simulink model "MicrogridControl"  (R2025b)
settings: Solver=VariableStepAuto  StartTime=0.0  StopTime=8  FixedStep=Ts  RelTol=1e-3
PreLoadFcn:
  | NormalOperation;
  | MicrogridControlParam;
undefined symbols (not defined in the file): base, bessModeInitial, bessSystem, bessVoltage, breakerStatus, DiscIntNeverNeededParam, ee_sli_rtmsupport, event, gcbh, generator, gflInverter, gfmInverter, Inertia, lineInductance, lineResistance, machine, plannedIsland, pmsm, powerLimit, powerQuality, PV, PVInverter, ref, resync, solar, solarInsolationChange, systemFrequency, Ts, windController, windSystem, windTurbine
libraries: nesl_utility x234, ee_lib x174, fl_lib x143, eeGeneralControl x137, simulink x78, eeTransforms x47, slpidlib x23, nesl_utility_internal x12, eePwmGenerator x9, eeSinusoidalMeasurementV2 x9, custom_lib x7, batteryecm_lib x6
(part 3 of 25)

== system MicrogridControl/Solar ==
  Constant1 : Constant  Value=298
  Constant2 : Constant  Value=0
  Constant3 : Constant  Value=0
  Constant4 : Constant
  Solar Plant Integrated : Subsystem  Variant=on  VariantControlMode=label  LabelModeActiveChoice=Detailed  mask(Solar){fidelity=Detailed, plantRating=PV.plantRating, Vac=PV.Vac, frequency=PV.frequency, iMaxPU=PVInverter.iMaxPU, efficiency=PV.converterEfficiency, baseVoltageDC=PV.baseVoltageDC, nParallel=112, nSeries=30, capacitance=PVInverter.capacitance, filterInductance=PVInverter.filterInductance, filterResistance=PVInverter.filterResistance, panelType=Poly-crystalline, panelRating=PV.panelRating, Isc=PV.Isc, Voc=PV.Voc, irradianceSTC=PV.irradianceSTC, temperatureSTC=PV.temperatureSTC, alpha=PV.alpha, beta=PV.beta, mode=Maximum power point tracking, converterFidelity=Average, fSw=PV.switchingFrequency}
      mask prompts: fidelity "Modeling Option"; plantRating "Solar Plant Rating (kW)"; Vac "Rated AC side voltage (phase-phase RMS) (V)"; frequency "Rated electrical frequency at AC side (Hz)"; iMaxPU "Maximum converter current (pu)"; efficiency "Converter Efficiency (%)"; baseVoltageDC "Voltage on DC side (V)"; nParallel "Number of panels in parallel"; nSeries "Number of panels in series"; capacitance "DC bus capacitance (F)"; filterInductance "Filter inductance (H)"; filterResistance "Filter series resistance (Ohm)"; panelType "Panel Type"; panelRating "Panel Rating (W)"; Isc "Short-circuit current (A)"; Voc "Open-circuit voltage (V)"; irradianceSTC "Irradiance at STC (W/m² )"; temperatureSTC "Temperature at STC (°K)"; alpha "Temperature co-efficient for current (A/°K)"; beta "Temperature co-efficient for voltage (V/°K)"; mode "Operating Mode"; converterFidelity "Converter Fidelity"; fSw "Switching Frequency (kHz)"
      mask help: This block models a Solar PV plant. The detailed variant models MPPT, voltage and current controllers. The simplified variant is based on Anderson's translational equations. Select simplified mode for faster simulation using fixed efficiency and rated power.
      settings: CopyFcn=set_param(gcbh,'LinkStatus','none');
      mask Help: web('SolarPlant.html')
      mask TypeOptions fidelity: Detailed | Simplified
      mask Callback fidelity: component.mask.fidelitySelection;
      mask TypeOptions nParallel: Detailed/PV Plant & Controller/PV Plant/nParallel
      mask TypeOptions nSeries: Detailed/PV Plant & Controller/PV Plant/nSeries
      mask TypeOptions panelType: Poly-crystalline | Mono-crystalline | Cadmium-Telluride | Others
      mask Callback panelType: component.mask.selectSolarPanelType;
      mask TypeOptions mode: Maximum power point tracking | Power reference
      mask Callback mode:
      | % choice = get_param(gcb,'mode');
      | % blockPath = [gcb,'/','Solar','/','Simplified','/','Solar_Plant'];
      | % blockHandle = get_param(blockPath, 'Handle');
      | % if strcmp(choice,'Maximum power point tracking')
      | %     set_param(blockPath,'modelling_option','ModellingOption.maximumPower');
      | % else
      | %     set_param(blockPath,'modelling_option','ModellingOption.powerReference');
      | % end
      mask TypeOptions converterFidelity: Detailed/PV Plant & Controller/PV Plant/converterFidelity
      mask Callback converterFidelity: component.mask.setSwitchingFrequency;
      mask TypeOptions fSw: Detailed/PV Plant & Controller/PV Plant/fSw
      mask DialogControl generalDetailed Prompt: General
      mask DialogControl cellDetailed Prompt: Solar Cell
      mask DialogControl partsCatalog Prompt: Click to choose from parts catalog
      mask DialogControl partsCatalog Callback: component.mask.openParamManager;
      mask DialogControl panelCalculation Prompt: Calculate number of panels
      mask DialogControl panelCalculation Callback: component.mask.setPanelNumber;
      mask DialogControl configureSolarCell Prompt: Edit Solar Cell Parameters
      mask DialogControl configureSolarCell Callback:
      | blockPath = [gcb,'/','Detailed','/','PV Plant & Controller','/','PV Plant','/','PV Array'];
      |     component.mask.openBlock(blockPath);
      mask DialogControl controllerDetailed Prompt: Solar PV Controller
      mask DialogControl configurePVController Prompt: Edit MPPT Controller
      mask DialogControl configurePVController Callback:
      | blockPath = [gcb,'/','Detailed','/','PV Plant & Controller','/','Controller','/','MPPT','/','Solar PV Controller'];
      |     component.mask.openBlock(blockPath);
      mask DialogControl configurePRefControl Prompt: Edit Power Reference Controller
      mask DialogControl configurePRefControl Callback:
      | blockPath = [gcb,'/','Detailed','/','PV Plant & Controller','/','Controller','/','Power Reference','/','Power Reference Controller'];
      |     component.mask.openBlock(blockPath);
      mask DialogControl cellSimplified Prompt: Solar Cell
      mask DialogControl converter Prompt: Converter
      mask DialogControl editConverter Prompt: Edit converter parameters
      mask DialogControl editConverter Callback:
      | converterFidelity = get_param(gcb,'converterFidelity');
      | blockPath = [gcb,'/','Detailed','/','PV Plant & Controller','/','PV Plant','/','Converter','/',converterFidelity,'/','Converter'];
      | component.mask.openBlock(blockPath);
      mask Display: image('solarPlant.png');
  Solar Plant Integrated1 : Subsystem  Variant=on  VariantControlMode=label  LabelModeActiveChoice=Detailed  mask(Solar){fidelity=Detailed, plantRating=PV.plantRating, Vac=PV.Vac, frequency=PV.frequency, iMaxPU=PVInverter.iMaxPU, efficiency=PV.converterEfficiency, baseVoltageDC=PV.baseVoltageDC, nParallel=112, nSeries=30, capacitance=PVInverter.capacitance, filterInductance=PVInverter.filterInductance, filterResistance=PVInverter.filterResistance, panelType=Poly-crystalline, panelRating=PV.panelRating, Isc=PV.Isc, Voc=PV.Voc, irradianceSTC=PV.irradianceSTC, temperatureSTC=PV.temperatureSTC, alpha=PV.alpha, beta=PV.beta, mode=Maximum power point tracking, converterFidelity=Average, fSw=PV.switchingFrequency}
      mask prompts: fidelity "Modeling Option"; plantRating "Solar Plant Rating (kW)"; Vac "Rated AC side voltage (phase-phase RMS) (V)"; frequency "Rated electrical frequency at AC side (Hz)"; iMaxPU "Maximum converter current (pu)"; efficiency "Converter Efficiency (%)"; baseVoltageDC "Voltage on DC side (V)"; nParallel "Number of panels in parallel"; nSeries "Number of panels in series"; capacitance "DC bus capacitance (F)"; filterInductance "Filter inductance (H)"; filterResistance "Filter series resistance (Ohm)"; panelType "Panel Type"; panelRating "Panel Rating (W)"; Isc "Short-circuit current (A)"; Voc "Open-circuit voltage (V)"; irradianceSTC "Irradiance at STC (W/m² )"; temperatureSTC "Temperature at STC (°K)"; alpha "Temperature co-efficient for current (A/°K)"; beta "Temperature co-efficient for voltage (V/°K)"; mode "Operating Mode"; converterFidelity "Converter Fidelity"; fSw "Switching Frequency (kHz)"
      mask help: This block models a Solar PV plant. The detailed variant models MPPT, voltage and current controllers. The simplified variant is based on Anderson's translational equations. Select simplified mode for faster simulation using fixed efficiency and rated power.
      settings: CopyFcn=set_param(gcbh,'LinkStatus','none');
      mask Help: web('SolarPlant.html')
      mask TypeOptions fidelity: Detailed | Simplified
      mask Callback fidelity: component.mask.fidelitySelection;
      mask TypeOptions nParallel: Detailed/PV Plant & Controller/PV Plant/nParallel
      mask TypeOptions nSeries: Detailed/PV Plant & Controller/PV Plant/nSeries
      mask TypeOptions panelType: Poly-crystalline | Mono-crystalline | Cadmium-Telluride | Others
      mask Callback panelType: component.mask.selectSolarPanelType;
      mask TypeOptions mode: Maximum power point tracking | Power reference
      mask Callback mode:
      | % choice = get_param(gcb,'mode');
      | % blockPath = [gcb,'/','Solar','/','Simplified','/','Solar_Plant'];
      | % blockHandle = get_param(blockPath, 'Handle');
      | % if strcmp(choice,'Maximum power point tracking')
      | %     set_param(blockPath,'modelling_option','ModellingOption.maximumPower');
      | % else
      | %     set_param(blockPath,'modelling_option','ModellingOption.powerReference');
      | % end
      mask TypeOptions converterFidelity: Detailed/PV Plant & Controller/PV Plant/converterFidelity
      mask Callback converterFidelity: component.mask.setSwitchingFrequency;
      mask TypeOptions fSw: Detailed/PV Plant & Controller/PV Plant/fSw
      mask DialogControl generalDetailed Prompt: General
      mask DialogControl cellDetailed Prompt: Solar Cell
      mask DialogControl partsCatalog Prompt: Click to choose from parts catalog
      mask DialogControl partsCatalog Callback: component.mask.openParamManager;
      mask DialogControl panelCalculation Prompt: Calculate number of panels
      mask DialogControl panelCalculation Callback: component.mask.setPanelNumber;
      mask DialogControl configureSolarCell Prompt: Edit Solar Cell Parameters
      mask DialogControl configureSolarCell Callback:
      | blockPath = [gcb,'/','Detailed','/','PV Plant & Controller','/','PV Plant','/','PV Array'];
      |     component.mask.openBlock(blockPath);
      mask DialogControl controllerDetailed Prompt: Solar PV Controller
      mask DialogControl configurePVController Prompt: Edit MPPT Controller
      mask DialogControl configurePVController Callback:
      | blockPath = [gcb,'/','Detailed','/','PV Plant & Controller','/','Controller','/','MPPT','/','Solar PV Controller'];
      |     component.mask.openBlock(blockPath);
      mask DialogControl configurePRefControl Prompt: Edit Power Reference Controller
      mask DialogControl configurePRefControl Callback:
      | blockPath = [gcb,'/','Detailed','/','PV Plant & Controller','/','Controller','/','Power Reference','/','Power Reference Controller'];
      |     component.mask.openBlock(blockPath);
      mask DialogControl cellSimplified Prompt: Solar Cell
      mask DialogControl converter Prompt: Converter
      mask DialogControl editConverter Prompt: Edit converter parameters
      mask DialogControl editConverter Callback:
      | converterFidelity = get_param(gcb,'converterFidelity');
      | blockPath = [gcb,'/','Detailed','/','PV Plant & Controller','/','PV Plant','/','Converter','/',converterFidelity,'/','Converter'];
      | component.mask.openBlock(blockPath);
      mask Display: image('solarPlant.png');
  Step1 : Step  Time=solarInsolationChange  Before=1000  After=800  SampleTime=0
  Transformer : Subsystem  Variant=on  VariantControlMode=label  LabelModeActiveChoice=Detailed  mask{fidelity=Detailed}
      mask prompts: fidelity "Modeling Option"
      mask TypeOptions fidelity: Detailed | Simplified
      mask Callback fidelity:
      | choice = get_param(gcb,'fidelity');
      | switch choice
      |     case 'Detailed'
      |         set_param(gcb, 'LabelModeActiveChoice', 'Detailed');
      |     case 'Simplified'
      |          set_param(gcb, 'LabelModeActiveChoice', 'Simplified');
      |     otherwise
      |         disp('Choose proper variant');
      | end
  Transformer1 : Subsystem  Variant=on  VariantControlMode=label  LabelModeActiveChoice=Detailed  mask{fidelity=Detailed}
      mask prompts: fidelity "Modeling Option"
      mask TypeOptions fidelity: Detailed | Simplified
      mask Callback fidelity:
      | choice = get_param(gcb,'fidelity');
      | switch choice
      |     case 'Detailed'
      |         set_param(gcb, 'LabelModeActiveChoice', 'Detailed');
      |     case 'Simplified'
      |          set_param(gcb, 'LabelModeActiveChoice', 'Simplified');
      |     otherwise
      |         disp('Choose proper variant');
      | end
  ~ : PMIOPort  Side=Left
  wires:
  Constant1/1 -> Solar Plant Integrated1/2(T), Solar Plant Integrated/2(T)
  Constant4/1 -> Solar Plant Integrated1/5(Mode), Solar Plant Integrated/5(Mode)
  Constant2/1 -> Solar Plant Integrated1/3(Pref), Solar Plant Integrated/3(Pref)
  Constant3/1 -> Solar Plant Integrated1/4(Qref), Solar Plant Integrated/4(Qref)
  Step1/1 -> Solar Plant Integrated1/1(Ir), Solar Plant Integrated/1(Ir)
  connections:
  Transformer/RConn1 -- Transformer1/RConn1 -- ~/RConn1
  Solar Plant Integrated/RConn1 -- Transformer/LConn1
  Solar Plant Integrated1/RConn1 -- Transformer1/LConn1

== system MicrogridControl/Subsystem ==
  Subsystem1 : Subsystem
      settings: PortSchema="{\"entries\":[{\"content\":{\"sides\":[{\"content\":{\"connectorIds\":[\"LConn1\"]},\"type\":\"ConnectorPlacement.EquallySpacedRectSide\",\"uuid\":\"0c8863a2-a78f-4a73-a820-c6aa5bdc2133\"},{\"content\":{\"connectorIds\":[\"RConn1\"],\"side\":\"RIGHT\"},\"type\":\"ConnectorPlacement.EquallySpacedRectSide\",\"uuid\":\"2028a368-e468-46fb-8c3f-9ce74e7f0a45\"},{\"content\":{\"side\":\"TOP\"},\"type\":\"ConnectorPlacement.EquallySpacedRectSide\",\"uuid\":\"1b144116-ac84-43c3-ac53-ab33c5b71658\"},{\"content\":{\"connectorIds\":[\"Out1\",\"Out2\"],\"side\":\"BOTTOM\"},\"type\":\"ConnectorPlacement.EquallySpacedRectSide\",\"uuid\":\"3e4d0e65-8f44-4e57-8d60-68941db834c2\"}]},\"type\":\"ConnectorPlacement.EquallySpacedConnector\",\"uuid\":\"a27c8f54-ed82-4619-aed8-d6cf5e2c28e1\"}],\"packageUris\":[\"http://schema.mathworks.com/mf0/Connector/R2020b\"],\"version\":\"1.0\"}"
      mask Display: image('measurements.png');
  Conn1 : PMIOPort  Side=Left
  Conn2 : PMIOPort  Port=2  Side=Right
  Bus Element Out : Outport  PortName=Solar  Element=P
  BusElementOut : Outport  PortName=Solar  Element=Q
  wires:
  Subsystem1/2(P) -> Bus Element Out/1  "Solar"
  Subsystem1/1(Q) -> BusElementOut/1  "Solar"
  connections:
  Conn1/RConn1 -- Subsystem1/RConn1
  Subsystem1/LConn1 -- Conn2/RConn1

== system MicrogridControl/Subsystem1 ==
  Circuit Breaker : Subsystem
  Constant : Constant  Value=breakerStatus.generator
  Subsystem9 : Subsystem
      settings: PortSchema="{\"entries\":[{\"content\":{\"sides\":[{\"content\":{\"connectorIds\":[\"LConn1\"]},\"type\":\"ConnectorPlacement.EquallySpacedRectSide\",\"uuid\":\"0c8863a2-a78f-4a73-a820-c6aa5bdc2133\"},{\"content\":{\"connectorIds\":[\"RConn1\"],\"side\":\"RIGHT\"},\"type\":\"ConnectorPlacement.EquallySpacedRectSide\",\"uuid\":\"2028a368-e468-46fb-8c3f-9ce74e7f0a45\"},{\"content\":{\"side\":\"TOP\"},\"type\":\"ConnectorPlacement.EquallySpacedRectSide\",\"uuid\":\"1b144116-ac84-43c3-ac53-ab33c5b71658\"},{\"content\":{\"connectorIds\":[\"Out1\",\"Out2\"],\"side\":\"BOTTOM\"},\"type\":\"ConnectorPlacement.EquallySpacedRectSide\",\"uuid\":\"3e4d0e65-8f44-4e57-8d60-68941db834c2\"}]},\"type\":\"ConnectorPlacement.EquallySpacedConnector\",\"uuid\":\"a27c8f54-ed82-4619-aed8-d6cf5e2c28e1\"}],\"packageUris\":[\"http://schema.mathworks.com/mf0/Connector/R2020b\"],\"version\":\"1.0\"}"
      mask Display: image('measurements.png');
  ~ : PMIOPort  Side=Left
  Conn2 : PMIOPort  Port=2  Side=Right
  Bus Element Out : Outport  PortName=Generator  Element=P
  BusElementOut : Outport  PortName=Generator  Element=Q
  wires:
  Subsystem9/2(P) -> Bus Element Out/1  "Diesel"
  Subsystem9/1(Q) -> BusElementOut/1  "Diesel"
  Constant/1 -> Circuit Breaker/1(BRK)
  connections:
  ~/RConn1 -- Circuit Breaker/LConn1
  Subsystem9/RConn1 -- Circuit Breaker/RConn1
  Conn2/RConn1 -- Subsystem9/LConn1

== system MicrogridControl/Subsystem10 ==
  In : PMIOPort  Side=Left
  Out : PMIOPort  Port=2  Side=Right
  connections:
  Out/RConn1 -- In/RConn1

== system MicrogridControl/Subsystem12 ==
  RLC (Three-Phase) : ee_lib/Passive/RLC Assemblies/RLC (Three-Phase)  port_option=ee.enum.threePhasePort.composite  component_structure=ee.enum.rlc.structure.SeriesRL  R=1e-2*10 Ohm  L=1e-6*10 H  C=1e-6 F  R_parasitic=0 Ohm  G_parasitic=0 1/Ohm  IL_specify=on  IL_priority=None  IL=[0, 0, 0] A  IL_nominal_specify=off  IL_nominal_value=1  IL_nominal_unit=A  VC_specify=off  VC_priority=High  VC=[0, 0, 0] V  VC_nominal_specify=off  VC_nominal_value=1  VC_nominal_unit=V
      settings: InternalSimscapePortConfiguration="{\"Bottom\":[],\"Left\":[{\"id\":\"N1\",\"label\":\"~1\",\"type\":\"foundation.electrical.three_phase\"}],\"Right\":[{\"id\":\"N2\",\"label\":\"~2\",\"type\":\"foundation.electrical.three_phase\"}],\"Top\":[]}"
  In : PMIOPort  Side=Left
  Out : PMIOPort  Port=2  Side=Right
  connections:
  RLC (Three-Phase)/LConn1 -- In/RConn1
  RLC (Three-Phase)/RConn1 -- Out/RConn1

== system MicrogridControl/Subsystem13 ==
  Electrical Reference : fl_lib/Electrical/Electrical Elements/Electrical Reference  Commented=on
  Subsystem : Subsystem
      settings: PortSchema="{\"entries\":[{\"content\":{\"sides\":[{\"content\":{\"connectorIds\":[\"LConn1\"]},\"type\":\"ConnectorPlacement.EquallySpacedRectSide\",\"uuid\":\"0c8863a2-a78f-4a73-a820-c6aa5bdc2133\"},{\"content\":{\"connectorIds\":[\"RConn1\"],\"side\":\"RIGHT\"},\"type\":\"ConnectorPlacement.EquallySpacedRectSide\",\"uuid\":\"2028a368-e468-46fb-8c3f-9ce74e7f0a45\"},{\"content\":{\"side\":\"TOP\"},\"type\":\"ConnectorPlacement.EquallySpacedRectSide\",\"uuid\":\"1b144116-ac84-43c3-ac53-ab33c5b71658\"},{\"content\":{\"connectorIds\":[\"Out1\",\"Out2\"],\"side\":\"BOTTOM\"},\"type\":\"ConnectorPlacement.EquallySpacedRectSide\",\"uuid\":\"3e4d0e65-8f44-4e57-8d60-68941db834c2\"}]},\"type\":\"ConnectorPlacement.EquallySpacedConnector\",\"uuid\":\"a27c8f54-ed82-4619-aed8-d6cf5e2c28e1\"}],\"packageUris\":[\"http://schema.mathworks.com/mf0/Connector/R2020b\"],\"version\":\"1.0\"}"
      mask Display: image('measurements.png');
  Two-Winding Transformer (Three-Phase)1 : ee_lib/Passive/Transformers/Two-Winding Transformer (Three-Phase)  Commented=on  SRated=5e6 A*V  FRated=60 Hz  Winding1Connection=ee.enum.windingconnection.Yg  VRated1=11000 V  Winding2Connection=ee.enum.windingconnection.Yg  VRated2=4160 V  CoreType=ee.enum.coretype.threelimb  pu_Rw1=0.01  pu_Rw2=0.01  leakage_reactance_option=ee.enum.transformer_leakage.include  pu_Xl1=0.05  pu_Xl2=0.05  magnetizing_resistance_option=ee.enum.transformer_magnetizingResistance.exclude  pu_Rm=500  magnetizing_reactance_option=ee.enum.transformer_magnetizingReactance.exclude  saturation_option=ee.enum.transformer_saturation.exclude  pu_Xm=500  current_data=[0, .002, 1, 2]  magnetic_flux_data=[0, 1.2, 1.5, 1.51]  pu_X0=0.5  i1_specify=off  i1_priority=None  i1=[0, 0, 0] A  i1_nominal_specify=off  i1_nominal_value=1  i1_nominal_unit=A  i2_specify=off  i2_priority=None  i2=[0, 0, 0] A  i2_nominal_specify=off  i2_nominal_value=1  i2_nominal_unit=A  phi_specify=off  phi_priority=None  phi=[0, 0, 0]  phi_nominal_specify=off  phi_nominal_value=1  phi_nominal_unit=1  power_dissipated_specify=off  power_dissipated_priority=None  power_dissipated=0 W  power_dissipated_nominal_specify=off  power_dissipated_nominal_value=1  power_dissipated_nominal_unit=W
      settings: InternalSimscapePortConfiguration="{\"Bottom\":[],\"Left\":[{\"id\":\"N1\",\"label\":\"~1\",\"type\":\"foundation.electrical.three_phase\"}],\"Right\":[{\"id\":\"N2\",\"label\":\"~2\",\"type\":\"foundation.electrical.three_phase\"}],\"Top\":[]}"
  Wye-Connected Load : ee_lib/Passive/RLC Assemblies/Wye-Connected Load  Commented=on  port_option=ee.enum.threePhasePort.composite  parameterization=ee.enum.rlc.parameterization.ratedpower  component_structure=ee.enum.rlc.structure.R  component_structure_PQ=ee.enum.rlc.structure.C  R=1 Ohm  L=1e-3 H  C=1e-6 F  VRated=6600 V  FRated=50 Hz  P=1e3 W  Qpos=1e2 A*V  Qneg=-0.4e6 A*V  R_parasitic=0 Ohm  G_parasitic=0 1/Ohm  R_parasitic_PQ=0 Ohm  G_parasitic_PQ=0 1/Ohm  Vmag0=0 V  Vang0=0 deg  Freq0=50 Hz  IL_specify=off  IL_priority=High  IL=[0, 0, 0] A  IL_nominal_specify=off  IL_nominal_value=1  IL_nominal_unit=A  VC_specify=off  VC_priority=High  VC=[0, 0, 0] V  VC_nominal_specify=off  VC_nominal_value=1  VC_nominal_unit=V
  Con : PMIOPort  Side=Left
  Conn2 : PMIOPort  Port=2  Side=Right
  Bus Element Out : Outport  PortName=BESS  Element=P
  BusElementOut : Outport  PortName=BESS  Element=Q
  wires:
  Subsystem/2(P) -> Bus Element Out/1  "BESS"
  Subsystem/1(Q) -> BusElementOut/1  "BESS"
  connections:
  Subsystem/LConn1 -- Wye-Connected Load/LConn1 -- Conn2/RConn1
  Con/RConn1 -- Subsystem/RConn1
  Electrical Reference/LConn1 -- Wye-Connected Load/RConn1

== system MicrogridControl/Subsystem14 ==
  Electrical Reference : fl_lib/Electrical/Electrical Elements/Electrical Reference
  Voltage Source (Three-Phase) : ee_lib/Sources/Voltage Source (Three-Phase)  vline_rms=gridVoltage V  shift=0 deg  freq=systemFrequency Hz  impedance_option=0  SShortCircuit=1e6 A*V  XR=15  R=0.01 Ohm  L=3.97e-4 H  harmonic_option=0  harmonic_orders=[5, 7, 11, 13]  harmonic_ratios=[.1, .1, .1, .1]  G_parasitic=0 1/Ohm  I_specify=off  I_priority=None  I=[0, 0, 0] A  I_nominal_specify=off  I_nominal_value=1  I_nominal_unit=A
  Conn2 : PMIOPort  Side=Left
  Conn1 : PMIOPort  Port=2  Side=Right
  connections:
  Voltage Source (Three-Phase)/LConn1 -- Conn2/RConn1 -- Electrical Reference/LConn1
  Conn1/RConn1 -- Voltage Source (Three-Phase)/RConn1

== system MicrogridControl/Subsystem15 ==
  BRK : Inport
  Circuit Breaker : Subsystem
  Gain : Gain  Gain=sqrt(3)/11000
  Gain1 : Gain  Gain=sqrt(3)/11000
  Grounded Neutral (Three-Phase) : ee_lib/Connectors & References/Grounded Neutral (Three-Phase)
  Grounded Neutral (Three-Phase)1 : ee_lib/Connectors & References/Grounded Neutral (Three-Phase)
  PS-Simulink Converter : nesl_utility/PS-Simulink Converter  PhysicalDomain=network_engine_domain  SubClassName=ps_output  LeftPortType=input  RightPortType=output  PseudoPeriodic=off  Frequencies=[]  VectorFormat=inherit  Unit=inherit  AffineConversion=off
  PS-Simulink Converter1 : nesl_utility/PS-Simulink Converter  PhysicalDomain=network_engine_domain  SubClassName=ps_output  LeftPortType=input  RightPortType=output  PseudoPeriodic=off  Frequencies=[]  VectorFormat=inherit  Unit=inherit  AffineConversion=off
  Phase Voltage Sensor (Three-Phase) : ee_lib/Sensors & Transducers/Phase Voltage Sensor (Three-Phase)
  Phase Voltage Sensor (Three-Phase)1 : ee_lib/Sensors & Transducers/Phase Voltage Sensor (Three-Phase)
  Scope : Scope
      settings: ActiveDisplayYMinimum=-1  ActiveDisplayYMaximum=1  DataLoggingVariableName=ScopeData25
  Scope1 : Scope  NumInputPorts=2
      settings: ActiveDisplayYMinimum=-2.9462782696915744  ActiveDisplayYMaximum=2.946278281849728  DataLoggingVariableName=ScopeData28
  Subsystem4 : Subsystem
      settings: PortSchema="{\"entries\":[{\"content\":{\"sides\":[{\"content\":{\"connectorIds\":[\"LConn1\"]},\"type\":\"ConnectorPlacement.EquallySpacedRectSide\",\"uuid\":\"0c8863a2-a78f-4a73-a820-c6aa5bdc2133\"},{\"content\":{\"connectorIds\":[\"RConn1\"],\"side\":\"RIGHT\"},\"type\":\"ConnectorPlacement.EquallySpacedRectSide\",\"uuid\":\"2028a368-e468-46fb-8c3f-9ce74e7f0a45\"},{\"content\":{\"side\":\"TOP\"},\"type\":\"ConnectorPlacement.EquallySpacedRectSide\",\"uuid\":\"1b144116-ac84-43c3-ac53-ab33c5b71658\"},{\"content\":{\"connectorIds\":[\"Out1\",\"Out2\"],\"side\":\"BOTTOM\"},\"type\":\"ConnectorPlacement.EquallySpacedRectSide\",\"uuid\":\"3e4d0e65-8f44-4e57-8d60-68941db834c2\"}]},\"type\":\"ConnectorPlacement.EquallySpacedConnector\",\"uuid\":\"a27c8f54-ed82-4619-aed8-d6cf5e2c28e1\"}],\"packageUris\":[\"http://schema.mathworks.com/mf0/Connector/R2020b\"],\"version\":\"1.0\"}"
      mask Display: image('measurements.png');
  Transformer : Subsystem  Variant=on  VariantControlMode=label  LabelModeActiveChoice=Detailed  mask{fidelity=Detailed}
      mask prompts: fidelity "Modeling Option"
      mask TypeOptions fidelity: Detailed | Simplified
      mask Callback fidelity:
      | choice = get_param(gcb,'fidelity');
      | switch choice
      |     case 'Detailed'
      |         set_param(gcb, 'LabelModeActiveChoice', 'Detailed');
      |     case 'Simplified'
      |          set_param(gcb, 'LabelModeActiveChoice', 'Simplified');
      |     otherwise
      |         disp('Choose proper variant');
      | end
  Conn1 : PMIOPort  Side=Left
  ~ : PMIOPort  Port=2  Side=Right
  Bus Element Out : Outport  PortName=Grid  Element=P
  BusElementOut : Outport  PortName=Grid  Element=Q
  BusElementOut3 : Outport  PortName=Grid  Element=gridVoltage
  BusElementOut4 : Outport  PortName=Grid  Element=PCCVoltage
  wires:
  Subsystem4/1(Q) -> BusElementOut/1  "Grid"
  Subsystem4/2(P) -> Bus Element Out/1  "Grid"
  BRK/1 -> Scope/1, Circuit Breaker/1(BRK)
  Gain1/1 -> Scope1/2, BusElementOut4/1
  PS-Simulink Converter1/1 -> Gain1/1
  Gain/1 -> Scope1/1, BusElementOut3/1
  PS-Simulink Converter/1 -> Gain/1
  connections:
  Subsystem4/RConn1 -- Transformer/LConn1
  Subsystem4/LConn1 -- Conn1/RConn1
  Circuit Breaker/LConn1 -- Phase Voltage Sensor (Three-Phase)/LConn1 -- Transformer/RConn1
  ~/RConn1 -- Circuit Breaker/RConn1 -- Phase Voltage Sensor (Three-Phase)1/LConn1
  Grounded Neutral (Three-Phase)/LConn1 -- Phase Voltage Sensor (Three-Phase)/RConn2
  PS-Simulink Converter/LConn1 -- Phase Voltage Sensor (Three-Phase)/RConn1
  PS-Simulink Converter1/LConn1 -- Phase Voltage Sensor (Three-Phase)1/RConn1
  Grounded Neutral (Three-Phase)1/LConn1 -- Phase Voltage Sensor (Three-Phase)1/RConn2

== system MicrogridControl/Subsystem3 ==
  Subsystem2 : Subsystem
      settings: PortSchema="{\"entries\":[{\"content\":{\"sides\":[{\"content\":{\"connectorIds\":[\"LConn1\"]},\"type\":\"ConnectorPlacement.EquallySpacedRectSide\",\"uuid\":\"0c8863a2-a78f-4a73-a820-c6aa5bdc2133\"},{\"content\":{\"connectorIds\":[\"RConn1\"],\"side\":\"RIGHT\"},\"type\":\"ConnectorPlacement.EquallySpacedRectSide\",\"uuid\":\"2028a368-e468-46fb-8c3f-9ce74e7f0a45\"},{\"content\":{\"side\":\"TOP\"},\"type\":\"ConnectorPlacement.EquallySpacedRectSide\",\"uuid\":\"1b144116-ac84-43c3-ac53-ab33c5b71658\"},{\"content\":{\"connectorIds\":[\"Out1\",\"Out2\"],\"side\":\"BOTTOM\"},\"type\":\"ConnectorPlacement.EquallySpacedRectSide\",\"uuid\":\"3e4d0e65-8f44-4e57-8d60-68941db834c2\"}]},\"type\":\"ConnectorPlacement.EquallySpacedConnector\",\"uuid\":\"a27c8f54-ed82-4619-aed8-d6cf5e2c28e1\"}],\"packageUris\":[\"http://schema.mathworks.com/mf0/Connector/R2020b\"],\"version\":\"1.0\"}"
      mask Display: image('measurements.png');
  Two-Winding Transformer (Three-Phase)4 : ee_lib/Passive/Transformers/Two-Winding Transformer (Three-Phase)  Commented=on  SRated=50e6 A*V  FRated=60 Hz  Winding1Connection=ee.enum.windingconnection.Yg  VRated1=11000 V  Winding2Connection=ee.enum.windingconnection.Yg  VRated2=690 V  CoreType=ee.enum.coretype.threelimb  pu_Rw1=0.01  pu_Rw2=0.01  leakage_reactance_option=ee.enum.transformer_leakage.include  pu_Xl1=0.05  pu_Xl2=0.05  magnetizing_resistance_option=ee.enum.transformer_magnetizingResistance.exclude  pu_Rm=500  magnetizing_reactance_option=ee.enum.transformer_magnetizingReactance.exclude  saturation_option=ee.enum.transformer_saturation.exclude  pu_Xm=500  current_data=[0, .002, 1, 2]  magnetic_flux_data=[0, 1.2, 1.5, 1.51]  pu_X0=0.5  i1_specify=off  i1_priority=None  i1=[0, 0, 0] A  i1_nominal_specify=off  i1_nominal_value=1  i1_nominal_unit=A  i2_specify=off  i2_priority=None  i2=[0, 0, 0] A  i2_nominal_specify=off  i2_nominal_value=1  i2_nominal_unit=A  phi_specify=off  phi_priority=None  phi=[0, 0, 0]  phi_nominal_specify=off  phi_nominal_value=1  phi_nominal_unit=1  power_dissipated_specify=off  power_dissipated_priority=None  power_dissipated=0 W  power_dissipated_nominal_specify=off  power_dissipated_nominal_value=1  power_dissipated_nominal_unit=W
      settings: InternalSimscapePortConfiguration="{\"Bottom\":[],\"Left\":[{\"id\":\"N1\",\"label\":\"~1\",\"type\":\"foundation.electrical.three_phase\"}],\"Right\":[{\"id\":\"N2\",\"label\":\"~2\",\"type\":\"foundation.electrical.three_phase\"}],\"Top\":[]}"
  Conn1 : PMIOPort  Side=Left
  Conn2 : PMIOPort  Port=2  Side=Right
  Bus Element Out : Outport  PortName=Load  Element=P
  BusElementOut : Outport  PortName=Load  Element=Q
  wires:
  Subsystem2/1(P) -> Bus Element Out/1  "Load"
  Subsystem2/2(Q) -> BusElementOut/1  "Load"
  connections:
  Subsystem2/RConn1 -- Conn2/RConn1
  Conn1/RConn1 -- Subsystem2/LConn1

== system MicrogridControl/Subsystem4 ==
  Electrical Reference : fl_lib/Electrical/Electrical Elements/Electrical Reference  Commented=on
  Subsystem3 : Subsystem
      settings: PortSchema="{\"entries\":[{\"content\":{\"sides\":[{\"content\":{\"connectorIds\":[\"LConn1\"]},\"type\":\"ConnectorPlacement.EquallySpacedRectSide\",\"uuid\":\"0c8863a2-a78f-4a73-a820-c6aa5bdc2133\"},{\"content\":{\"connectorIds\":[\"RConn1\"],\"side\":\"RIGHT\"},\"type\":\"ConnectorPlacement.EquallySpacedRectSide\",\"uuid\":\"2028a368-e468-46fb-8c3f-9ce74e7f0a45\"},{\"content\":{\"side\":\"TOP\"},\"type\":\"ConnectorPlacement.EquallySpacedRectSide\",\"uuid\":\"1b144116-ac84-43c3-ac53-ab33c5b71658\"},{\"content\":{\"connectorIds\":[\"Out1\",\"Out2\"],\"side\":\"BOTTOM\"},\"type\":\"ConnectorPlacement.EquallySpacedRectSide\",\"uuid\":\"3e4d0e65-8f44-4e57-8d60-68941db834c2\"}]},\"type\":\"ConnectorPlacement.EquallySpacedConnector\",\"uuid\":\"a27c8f54-ed82-4619-aed8-d6cf5e2c28e1\"}],\"packageUris\":[\"http://schema.mathworks.com/mf0/Connector/R2020b\"],\"version\":\"1.0\"}"
      mask Display: image('measurements.png');
  Wye-Connected Load : ee_lib/Passive/RLC Assemblies/Wye-Connected Load  Commented=on  port_option=ee.enum.threePhasePort.composite  parameterization=ee.enum.rlc.parameterization.ratedpower  component_structure=ee.enum.rlc.structure.R  component_structure_PQ=ee.enum.rlc.structure.C  R=1 Ohm  L=1e-3 H  C=1e-6 F  VRated=6600 V  FRated=50 Hz  P=1e3 W  Qpos=1e2 A*V  Qneg=-0.4e6 A*V  R_parasitic=0 Ohm  G_parasitic=0 1/Ohm  R_parasitic_PQ=0 Ohm  G_parasitic_PQ=0 1/Ohm  Vmag0=0 V  Vang0=0 deg  Freq0=50 Hz  IL_specify=off  IL_priority=High  IL=[0, 0, 0] A  IL_nominal_specify=off  IL_nominal_value=1  IL_nominal_unit=A  VC_specify=off  VC_priority=High  VC=[0, 0, 0] V  VC_nominal_specify=off  VC_nominal_value=1  VC_nominal_unit=V
  Conn1 : PMIOPort  Side=Left
  Conn2 : PMIOPort  Port=2  Side=Right
  Bus Element Out : Outport  PortName=Wind  Element=P
  BusElementOut : Outport  PortName=Wind  Element=Q
  wires:
  Subsystem3/2(P) -> Bus Element Out/1  "Wind"
  Subsystem3/1(Q) -> BusElementOut/1  "Wind"
  connections:
  Conn1/RConn1 -- Subsystem3/RConn1
  Subsystem3/LConn1 -- Wye-Connected Load/LConn1 -- Conn2/RConn1
  Electrical Reference/LConn1 -- Wye-Connected Load/RConn1

== system MicrogridControl/Subsystem5 ==
  RLC (Three-Phase) : ee_lib/Passive/RLC Assemblies/RLC (Three-Phase)  port_option=ee.enum.threePhasePort.composite  component_structure=ee.enum.rlc.structure.SeriesRL  R=lineResistance Ohm  L=lineInductance H  C=1e-6 F  R_parasitic=0 Ohm  G_parasitic=0 1/Ohm  IL_specify=on  IL_priority=None  IL=[0, 0, 0] A  IL_nominal_specify=off  IL_nominal_value=1  IL_nominal_unit=A  VC_specify=off  VC_priority=High  VC=[0, 0, 0] V  VC_nominal_specify=off  VC_nominal_value=1  VC_nominal_unit=V
      settings: InternalSimscapePortConfiguration="{\"Bottom\":[],\"Left\":[{\"id\":\"N1\",\"label\":\"~1\",\"type\":\"foundation.electrical.three_phase\"}],\"Right\":[{\"id\":\"N2\",\"label\":\"~2\",\"type\":\"foundation.electrical.three_phase\"}],\"Top\":[]}"
  In : PMIOPort  Side=Left
  Out : PMIOPort  Port=2  Side=Right
  connections:
  RLC (Three-Phase)/LConn1 -- In/RConn1
  RLC (Three-Phase)/RConn1 -- Out/RConn1

== system MicrogridControl/Subsystem6 ==
  RLC (Three-Phase) : ee_lib/Passive/RLC Assemblies/RLC (Three-Phase)  port_option=ee.enum.threePhasePort.composite  component_structure=ee.enum.rlc.structure.SeriesRL  R=lineResistance Ohm  L=lineInductance H  C=1e-6 F  R_parasitic=0 Ohm  G_parasitic=0 1/Ohm  IL_specify=on  IL_priority=None  IL=[0, 0, 0] A  IL_nominal_specify=off  IL_nominal_value=1  IL_nominal_unit=A  VC_specify=off  VC_priority=High  VC=[0, 0, 0] V  VC_nominal_specify=off  VC_nominal_value=1  VC_nominal_unit=V
      settings: InternalSimscapePortConfiguration="{\"Bottom\":[],\"Left\":[{\"id\":\"N1\",\"label\":\"~1\",\"type\":\"foundation.electrical.three_phase\"}],\"Right\":[{\"id\":\"N2\",\"label\":\"~2\",\"type\":\"foundation.electrical.three_phase\"}],\"Top\":[]}"
  In : PMIOPort  Side=Left
  Out : PMIOPort  Port=2  Side=Right
  connections:
  RLC (Three-Phase)/LConn1 -- In/RConn1
  RLC (Three-Phase)/RConn1 -- Out/RConn1

== system MicrogridControl/Subsystem7 ==
  RLC (Three-Phase) : ee_lib/Passive/RLC Assemblies/RLC (Three-Phase)  port_option=ee.enum.threePhasePort.composite  component_structure=ee.enum.rlc.structure.SeriesRL  R=lineResistance Ohm  L=lineInductance H  C=1e-6 F  R_parasitic=0 Ohm  G_parasitic=0 1/Ohm  IL_specify=on  IL_priority=None  IL=[0, 0, 0] A  IL_nominal_specify=off  IL_nominal_value=1  IL_nominal_unit=A  VC_specify=off  VC_priority=High  VC=[0, 0, 0] V  VC_nominal_specify=off  VC_nominal_value=1  VC_nominal_unit=V
      settings: InternalSimscapePortConfiguration="{\"Bottom\":[],\"Left\":[{\"id\":\"N1\",\"label\":\"~1\",\"type\":\"foundation.electrical.three_phase\"}],\"Right\":[{\"id\":\"N2\",\"label\":\"~2\",\"type\":\"foundation.electrical.three_phase\"}],\"Top\":[]}"
  In : PMIOPort  Side=Left
  Out : PMIOPort  Port=2  Side=Right
  connections:
  RLC (Three-Phase)/LConn1 -- In/RConn1
  RLC (Three-Phase)/RConn1 -- Out/RConn1

== system MicrogridControl/Subsystem8 ==
  RLC (Three-Phase) : ee_lib/Passive/RLC Assemblies/RLC (Three-Phase)  port_option=ee.enum.threePhasePort.composite  component_structure=ee.enum.rlc.structure.SeriesRL  R=lineResistance Ohm  L=lineInductance H  C=1e-6 F  R_parasitic=0 Ohm  G_parasitic=0 1/Ohm  IL_specify=on  IL_priority=None  IL=[0, 0, 0] A  IL_nominal_specify=off  IL_nominal_value=1  IL_nominal_unit=A  VC_specify=off  VC_priority=High  VC=[0, 0, 0] V  VC_nominal_specify=off  VC_nominal_value=1  VC_nominal_unit=V
      settings: InternalSimscapePortConfiguration="{\"Bottom\":[],\"Left\":[{\"id\":\"N1\",\"label\":\"~1\",\"type\":\"foundation.electrical.three_phase\"}],\"Right\":[{\"id\":\"N2\",\"label\":\"~2\",\"type\":\"foundation.electrical.three_phase\"}],\"Top\":[]}"
  In : PMIOPort  Side=Left
  Out : PMIOPort  Port=2  Side=Right
  connections:
  RLC (Three-Phase)/LConn1 -- In/RConn1
  RLC (Three-Phase)/RConn1 -- Out/RConn1
